simulink model "controller_lqr"  (R2015b)
settings: Solver=ode3  StartTime=0  StopTime=inf  FixedStep=sampleTime_qcsim  MaxStep=0.1  RelTol=1e-3
InitFcn:
  | % load parameters of the default quadrotor
  | disp('Quadrotor parameters loaded by InitFcn')
  | paramsControl %load mdl_quadcopter as well!
values from neighbouring files (symbols this model uses):
  controlHelperParams =     [linsys1.mat]
  quad =     [linsys1.mat]
  quadEDT =     [linsys1.mat]
settings Model: Creator=corkep  LastModifiedBy=student
settings DataIOCC: LimitDataPoints=off  SaveFormat=StructureWithTime  SignalLoggingSaveFormat=ModelDataLogs  SignalLogging=off  DSMLogging=off
settings OptimizationCC: ExpressionDepthLimit=2147483647  OptimizeModelRefInitCode=on  LifeSpan=1
settings DebuggingCC: UnderspecifiedInitializationDetection=Classic  MergeDetectMultiDrivingBlocksExec=none  SolverPrmCheckMsg=warning  FcnCallInpInsideContextMsg=UseLocalSettings  StateNameClashWarn=warning
settings HardwareCC: ProdBitPerPointer=32  ProdLargestAtomicFloat=None  ProdIntDivRoundTo=Undefined  ProdEndianess=Unspecified  ProdWordSize=32  ProdHWDeviceType=32-bit Generic  TargetBitPerLong=64  TargetBitPerPointer=64  TargetLongLongMode=on  TargetIntDivRoundTo=Zero  TargetEndianess=LittleEndian  TargetWordSize=64  TargetHWDeviceType=MATLAB Host  ProdEqTarget=off
settings RTWCC: SystemTargetFile=ert_shrlib.tlc  GenCodeOnly=on  MakeCommand="make_rtw OPTS=\"-DDEFAULT_BUFFER_SIZE=4600\""  GenerateMakefile=off  TemplateMakefile=ert_default_tmf  Description=Embedded Coder (host-based shared library target)  BuildConfiguration=Faster Runs  RTWCompilerOptimization=on
settings CodeAppCC: IgnoreCustomStorageClasses=off
settings STFCustomTargetCC: GenerateSampleERTMain=on  ParMdlRefBuildCompliant=on  CompOptLevelCompliant=on  ConcurrentExecutionCompliant=off  IncludeMdlTerminateFcn=off  GeneratePreprocessorConditionals=Use local settings  CombineOutputUpdateFcns=on  ERTCustomFileBanners=on  MatFileLogging=on  MultiInstanceERTCode=on  CodeInterfacePackaging=Reusable function  SupportContinuousTime=off  SupportNonInlinedSFcns=off  MATLABClassNameForMDSCustomization=Simulink.SoftwareTarget.ERTCustomization  ModelStepFunctionPrototypeControlCompliant=on  CPPClassGenCompliant=off  GRTInterface=off  UseToolchainInfoCompliant=on  SystemTargetFile=ert_shrlib.tlc
settings ERTTargetCC: GenerateSampleERTMain=on  ConcurrentExecutionCompliant=off  IncludeMdlTerminateFcn=off  ERTFirstTimeCompliant=off  MatFileLogging=on  MultiInstanceERTCode=on  CodeInterfacePackaging=Reusable function  CPPClassGenCompliant=off  MultiInstanceErrorCode=Warning  ERTCustomFileTemplate=example_file_process.tlc
settings ConfigComp: CovModelRefEnable=Off  CovSFcnEnable=off

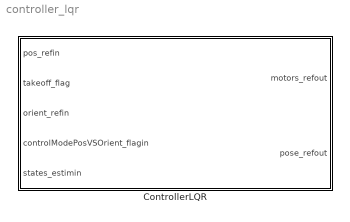
== system controller_lqr ==
  ControllerLQR : Subsystem  TreatAsAtomicUnit=on

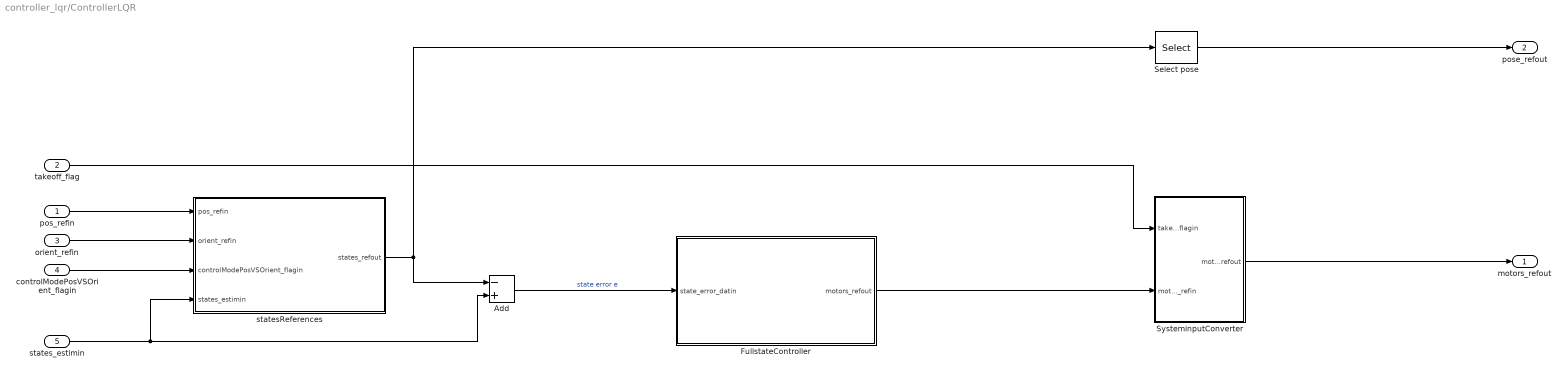
== system controller_lqr/ControllerLQR ==
  pos_refin : Inport
  takeoff_flag : Inport  Port=2
  orient_refin : Inport  Port=3
  controlModePosVSOrient_flagin : Inport  Port=4
  states_estimin : Inport  Port=5
  Add : Sum  Inputs=-+
  FullstateController : Subsystem
  Select pose : Selector  InputPortWidth=12  IndexOptions=Index vector (dialog)  Indices=[1:6]  OutputSizes=1
  SysteminputConverter : Subsystem
  statesReferences : Subsystem
  motors_refout : Outport
  pose_refout : Outport  Port=2
  wires:
  Select pose/1 -> pose_refout/1
  statesReferences/1(states_refout) -> Add/1, Select pose/1
  controlModePosVSOrient_flagin/1 -> statesReferences/3(controlModePosVSOrient_flagin)
  states_estimin/1 -> statesReferences/4(states_estimin), Add/2
  orient_refin/1 -> statesReferences/2(orient_refin)
  pos_refin/1 -> statesReferences/1(pos_refin)
  Add/1 -> FullstateController/1(state_error_datin)  "state error e"
  FullstateController/1(motors_refout) -> SysteminputConverter/2(motors_refin)
  SysteminputConverter/1(motors_refout) -> motors_refout/1
  takeoff_flag/1 -> SysteminputConverter/1(takeoffphase_flagin)

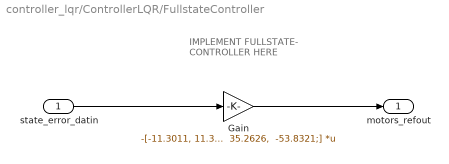
== system controller_lqr/ControllerLQR/FullstateController ==
  note: IMPLEMENT FULLSTATE-
      | CONTROLLER HERE
  state_error_datin : Inport
  Gain : Gain  Gain=|  Multiplication=Matrix(K*u) (u vector)
      | -[-11.3011, 11.3011,  -11.3011,  -47.0877,  118.6064,  117.6892,  -15.5707,   15.5113,  -24.4160 ,  34.5955,   35.2626,  -53.8321;
      |    11.3011,   11.3011,   11.3011,  -47.0877, -118.6064,  117.6892,   15.5707,   15.5113,   24.4160,   34.5955,  -35.2626,  -53.8321;
      |    11.3011,  -11.3011,  -11.3011,  -47.0877, -118.6064, -117.6892,   15.5707,  -15.5113,  -24.4160,  -34.5955,  -35.2626,  -53.8321;
      |   -11.3011,  -11.3011,   11.3011,  -47.0877,  118.6064, -117.6892,  -15.5707,  -15.5113,   24.4160,  -34.5955,   35.2626,  -53.8321;]
  motors_refout : Outport
  wires:
  state_error_datin/1 -> Gain/1
  Gain/1 -> motors_refout/1

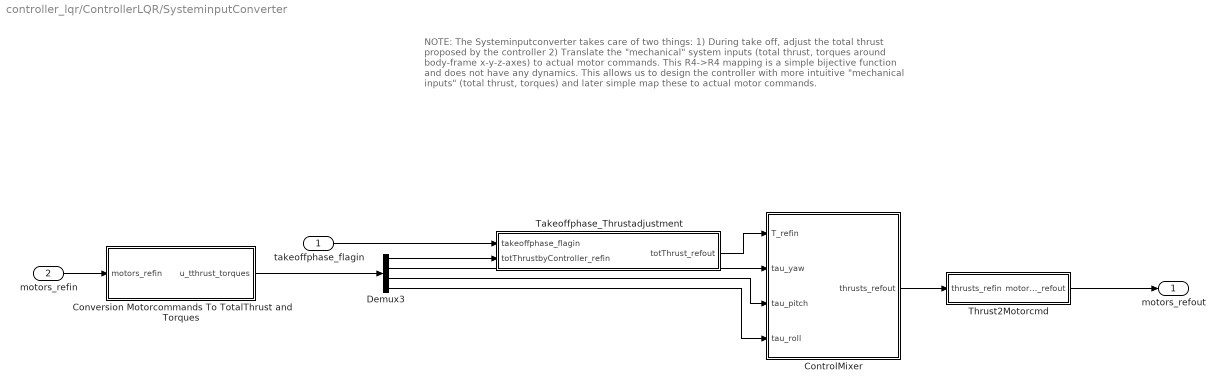
== system controller_lqr/ControllerLQR/SysteminputConverter ==
  note: NOTE: The Systeminputconverter takes care of two things:
      | 1) During take off, adjust the total thrust proposed by the controller
      | 2) Translate the "mechanical" system inputs (total thrust, torques around body-frame x-y-z-axes) to actual motor commands.
      | This R4->R4 mapping is a simple bijective function and does not have any dynamics. This allows us to design the controller with more intuitive "mechanical inputs" (total thrust, torques) and later simple map these to actual motor commands.
  takeoffphase_flagin : Inport
  motors_refin : Inport  Port=2
  ControlMixer : Subsystem
  Conversion Motorcommands To TotalThrust and Torques : Subsystem
  Demux3 : Demux
  Takeoffphase_Thrustadjustment : Subsystem
  Thrust2Motorcmd : Subsystem
  motors_refout : Outport
  wires:
  takeoffphase_flagin/1 -> Takeoffphase_Thrustadjustment/1(takeoffphase_flagin)
  Takeoffphase_Thrustadjustment/1(totThrust_refout) -> ControlMixer/1(T_refin)
  Demux3/1 -> Takeoffphase_Thrustadjustment/2(totThrustbyController_refin)
  Demux3/4 -> ControlMixer/4(tau_roll)
  Demux3/3 -> ControlMixer/3(tau_pitch)
  Demux3/2 -> ControlMixer/2(tau_yaw)
  ControlMixer/1(thrusts_refout) -> Thrust2Motorcmd/1(thrusts_refin)
  Thrust2Motorcmd/1(motors_refout) -> motors_refout/1
  motors_refin/1 -> Conversion Motorcommands To TotalThrust and Torques/1(motors_refin)
  Conversion Motorcommands To TotalThrust and Torques/1(u_tthrust_torques) -> Demux3/1

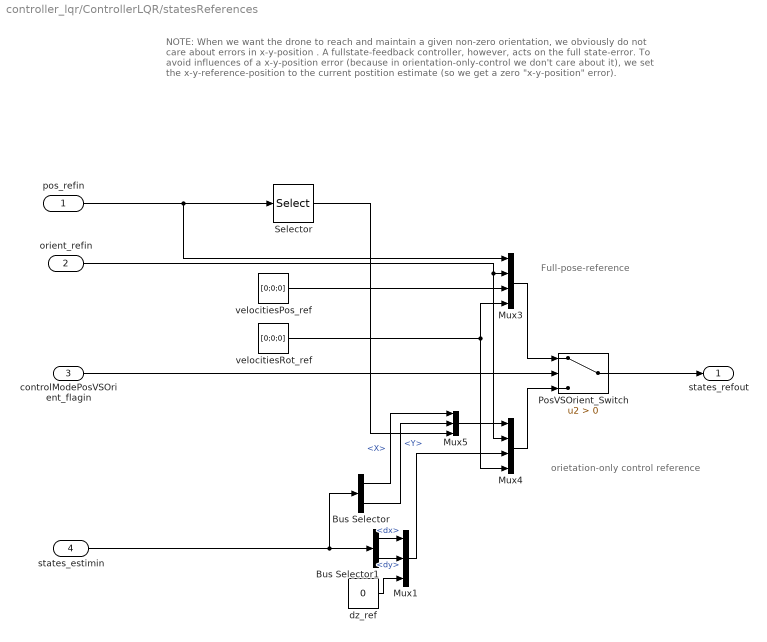
== system controller_lqr/ControllerLQR/statesReferences ==
  note: orietation-only control reference
  note: Full-pose-reference
  note: NOTE: When we want the drone to reach and maintain a given non-zero orientation,
      | we obviously do not care about errors in x-y-position . A fullstate-feedback controller, however, acts
      | on the full state-error. To avoid influences of a x-y-position error (because in orientation-only-control we don't care about it),
      | we set the x-y-reference-position to the current postition estimate (so we get a zero "x-y-position" error).
  pos_refin : Inport
  orient_refin : Inport  Port=2
  controlModePosVSOrient_flagin : Inport  Port=3
  states_estimin : Inport  Port=4
  Bus Selector : BusSelector  OutputSignals=X,Y
  Bus Selector1 : BusSelector  OutputSignals=dx,dy
  Mux1 : Mux  Inputs=3
  Mux3 : Mux
  Mux4 : Mux
  Mux5 : Mux  Inputs=3
  PosVSOrient_Switch : Switch  Criteria=u2 > Threshold
  Selector : Selector  InputPortWidth=3  IndexOptions=Index vector (dialog)  Indices=[3]  OutputSizes=1
  dz_ref : Constant  Value=0
  velocitiesPos_ref : Constant  Value=[0;0;0]
  velocitiesRot_ref : Constant  Value=[0;0;0]
  states_refout : Outport
  wires:
  dz_ref/1 -> Mux1/3
  Mux1/1 -> Mux4/3
  Bus Selector1/2 -> Mux1/2  "<dy>"
  Bus Selector1/1 -> Mux1/1  "<dx>"
  Mux5/1 -> Mux4/1
  Mux4/1 -> PosVSOrient_Switch/3
  Bus Selector/2 -> Mux5/2  "<Y>"
  Bus Selector/1 -> Mux5/1  "<X>"
  Mux3/1 -> PosVSOrient_Switch/1
  controlModePosVSOrient_flagin/1 -> PosVSOrient_Switch/2
  Selector/1 -> Mux5/3
  PosVSOrient_Switch/1 -> states_refout/1
  velocitiesRot_ref/1 -> Mux4/4, Mux3/4
  velocitiesPos_ref/1 -> Mux3/3
  states_estimin/1 -> Bus Selector/1, Bus Selector1/1
  orient_refin/1 -> Mux4/2, Mux3/2
  pos_refin/1 -> Mux3/1, Selector/1

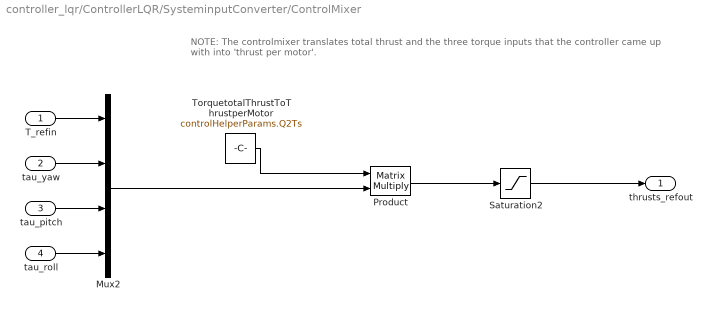
== system controller_lqr/ControllerLQR/SysteminputConverter/ControlMixer ==
  note: NOTE: The controlmixer translates total thrust and the three torque inputs that the controller came up with into 'thrust per motor'.
  T_refin : Inport
  tau_yaw : Inport  Port=2
  tau_pitch : Inport  Port=3
  tau_roll : Inport  Port=4
  Mux2 : Mux
  Product : Product  Multiplication=Matrix(*)  RndMeth=Zero
  Saturation2 : Saturate  UpperLimit=-0.05*controlHelperParams.motorsThrustperMotor_max  LowerLimit=-controlHelperParams.motorsThrustperMotor_max
  TorquetotalThrustToThrustperMotor : Constant  Value=controlHelperParams.Q2Ts
  thrusts_refout : Outport
  wires:
  tau_roll/1 -> Mux2/4
  tau_pitch/1 -> Mux2/3
  tau_yaw/1 -> Mux2/2
  T_refin/1 -> Mux2/1
  Product/1 -> Saturation2/1
  TorquetotalThrustToThrustperMotor/1 -> Product/1
  Mux2/1 -> Product/2
  Saturation2/1 -> thrusts_refout/1

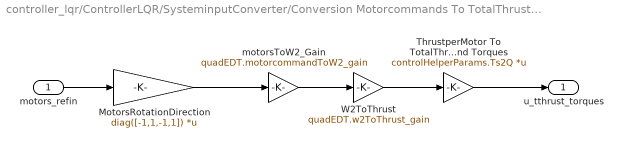
== system controller_lqr/ControllerLQR/SysteminputConverter/Conversion Motorcommands To TotalThrust and Torques ==
  motors_refin : Inport
  MotorsRotationDirection : Gain  Gain=diag([-1,1,-1,1])  Multiplication=Matrix(K*u)
  ThrustperMotor To TotalThrust and Torques : Gain  Gain=controlHelperParams.Ts2Q  Multiplication=Matrix(K*u)
  W2ToThrust : Gain  Gain=quadEDT.w2ToThrust_gain
  motorsToW2_Gain : Gain  Gain=quadEDT.motorcommandToW2_gain
  u_tthrust_torques : Outport
  wires:
  ThrustperMotor To TotalThrust and Torques/1 -> u_tthrust_torques/1
  motors_refin/1 -> MotorsRotationDirection/1
  W2ToThrust/1 -> ThrustperMotor To TotalThrust and Torques/1
  motorsToW2_Gain/1 -> W2ToThrust/1
  MotorsRotationDirection/1 -> motorsToW2_Gain/1

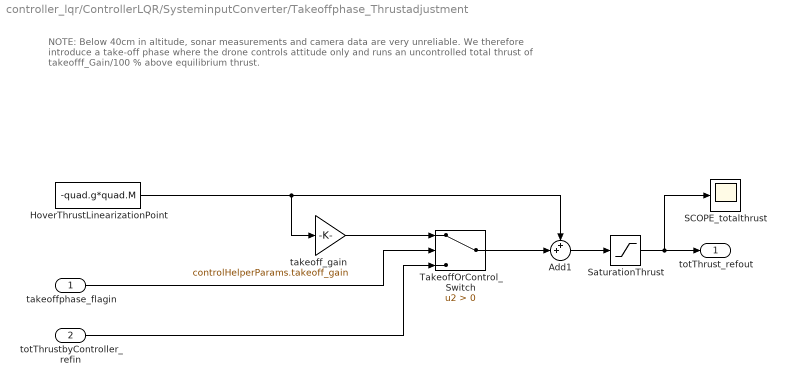
== system controller_lqr/ControllerLQR/SysteminputConverter/Takeoffphase_Thrustadjustment ==
  note: NOTE: Below 40cm in altitude, sonar measurements and camera data are very unreliable.
      | We therefore introduce a take-off phase where the drone controls attitude only and runs an uncontrolled total thrust of takeofff_Gain/100  % above equilibrium thrust.
  takeoffphase_flagin : Inport
  totThrustbyController_refin : Inport  Port=2
  Add1 : Sum  Inputs=++|
  HoverThrustLinearizationPoint : Constant  Value=-quad.g*quad.M
  "SCOPE_totalthrust " : Scope
  SaturationThrust : Saturate  UpperLimit=controlHelperParams.totalThrust_maxRelative*controlHelperParams.motorsThrustperMotor_max*4  LowerLimit=-controlHelperParams.totalThrust_maxRelative*controlHelperParams.motorsThrustperMotor_max*4
  TakeoffOrControl_Switch : Switch  Criteria=u2 > Threshold
  takeoff_gain : Gain  Gain=controlHelperParams.takeoff_gain
  totThrust_refout : Outport
  wires:
  takeoffphase_flagin/1 -> TakeoffOrControl_Switch/2
  SaturationThrust/1 -> totThrust_refout/1, "SCOPE_totalthrust "/1
  TakeoffOrControl_Switch/1 -> Add1/2
  takeoff_gain/1 -> TakeoffOrControl_Switch/1
  HoverThrustLinearizationPoint/1 -> Add1/1, takeoff_gain/1
  totThrustbyController_refin/1 -> TakeoffOrControl_Switch/3
  Add1/1 -> SaturationThrust/1

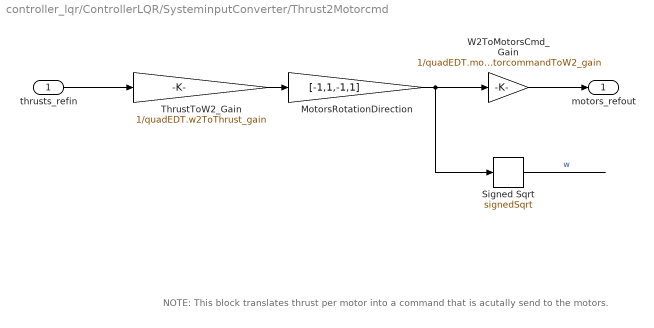
== system controller_lqr/ControllerLQR/SysteminputConverter/Thrust2Motorcmd ==
  note: NOTE: This block translates thrust per motor into a command that is acutally send to the motors.
  thrusts_refin : Inport
  MotorsRotationDirection : Gain  Gain=[-1,1,-1,1]
  Signed Sqrt : Sqrt  Operator=signedSqrt  SaturateOnIntegerOverflow=on
  ThrustToW2_Gain : Gain  Gain=1/quadEDT.w2ToThrust_gain
  W2ToMotorsCmd_Gain : Gain  Gain=1/quadEDT.motorcommandToW2_gain
  motors_refout : Outport
  wires:
  MotorsRotationDirection/1 -> W2ToMotorsCmd_Gain/1, Signed Sqrt/1
  Signed Sqrt/1 -> ?  "w"
  W2ToMotorsCmd_Gain/1 -> motors_refout/1
  thrusts_refin/1 -> ThrustToW2_Gain/1
  ThrustToW2_Gain/1 -> MotorsRotationDirection/1
